simulink model "PCM"  (R2023a)
settings: Solver=VariableStepAuto  StartTime=0.0  StopTime=1  RelTol=1e-3
undefined symbols (not defined in the file): comm, constellation
libraries: simulink x2, dspquant2 x2, dspfdesign x1, commutil2 x1, dspsrcs4 x1, dspsigops x1
settings Model: NumberOfSteps=10  Creator=mluser  LastModifiedBy=mluser

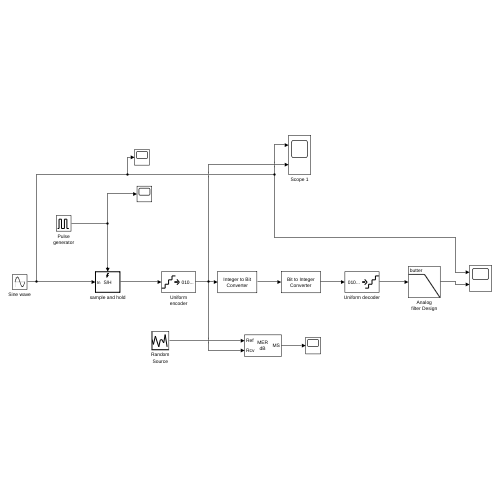
[thumbnail: Simulink's stored preview of the top-level diagram]
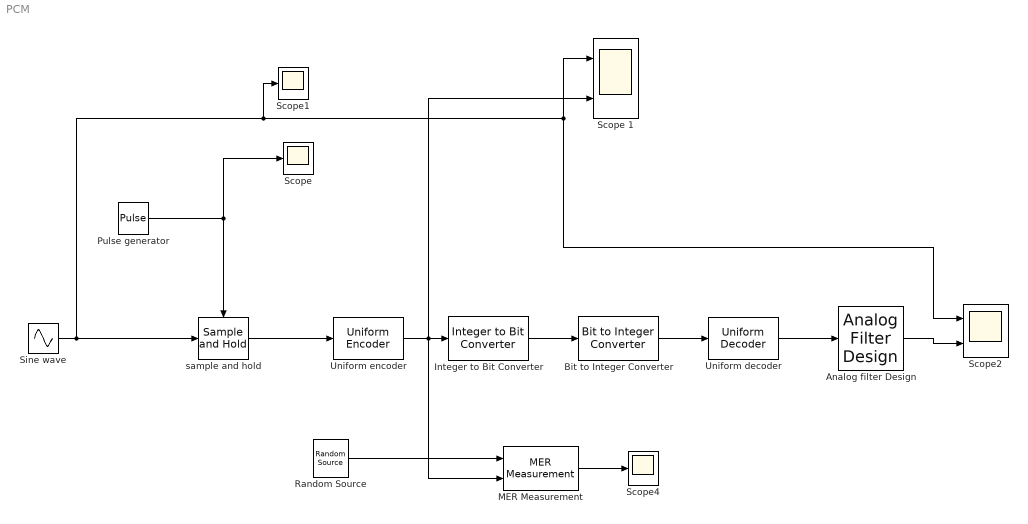
== system PCM ==
  Analog filter Design : dspfdesign/Analog Filter Design  method=Butterworth  filttype=Lowpass  N=8  Wlo=2*pi*2  Whi=80  Rp=2  Rs=40
  Bit to Integer Converter : simulink/Logic and Bit Operations/Bit to Integer Converter  nbits=3  bitOrder=MSB first  signedOutputValues=Signed  outDtype=Inherit via internal rule  outDtypeSigned=Inherit via internal rule
  Integer to Bit Converter : simulink/Logic and Bit Operations/Integer to Bit Converter  nbits=3  signedInputValues=Signed  bitOrder=MSB first  outDtype=Inherit via internal rule
  MER Measurement : commutil2/MER Measurement  ReferenceSignalSource=Input port  ReferenceConstellation=constellation( comm.QPSKModulator )  MeasurementIntervalSource=Input length  MeasurementInterval=100  AveragingDimensions=1  MinimumMEROutputPort=off  XPercentileMEROutputPort=off  XPercentileValue=95  SymbolCountOutputPort=off  SimulateUsing=Interpreted execution
  Pulse generator : DiscretePulseGenerator  PulseType=Time based  Amplitude=5  Period=1/20  PulseWidth=50
  Random Source : dspsrcs4/Random Source  SrcType=Gaussian  NormMethod=Ziggurat  CltLength=12  MinVal=0  MaxVal=1  MeanVal=0  VarVal=1  RepMode=Not repeatable  rawSeed=1  IsInherit=off  SampMode=Discrete  SampTime=1  SampFrame=1  DataType=Double  OutComplex=Real  OutputFrames=off
  Scope : Scope
  Scope 1 : Scope  NumInputPorts=2
  Scope1 : Scope
  Scope2 : Scope  NumInputPorts=2
  Scope4 : Scope
  Sine wave : Sin  Amplitude=5  Frequency=2*pi*2  SampleTime=0
  Uniform encoder : dspquant2/Uniform Encoder  peak=5  bits=3  otype=Signed integer
  Uniform decoder : dspquant2/Uniform Decoder  peak=5  bits=3  overflowMode=Saturate  otype=Double
  sample and hold : dspsigops/Sample and Hold  trig=Rising edge  initCond=0  latchinput=off
  wires:
  Sine wave/1 -> Scope1/1, Scope2/1, Scope 1/1, sample and hold/1
  sample and hold/1 -> Uniform encoder/1
  Uniform encoder/1 -> Scope 1/2, MER Measurement/2, Integer to Bit Converter/1
  Integer to Bit Converter/1 -> Bit to Integer Converter/1
  Bit to Integer Converter/1 -> Uniform decoder/1
  Uniform decoder/1 -> Analog filter Design/1
  Analog filter Design/1 -> Scope2/2
  Pulse generator/1 -> Scope/1, sample and hold/Trigger
  Random Source/1 -> MER Measurement/1
  MER Measurement/1 -> Scope4/1
